simulink model "Two_D_Maps"  (R2020a)
settings: Solver=VariableStepAuto  StartTime=0.0  StopTime=inf  RelTol=1e-3
PostLoadFcn:
  | data1=xlsread('performancemaps','VE');
  | rpm1=data1(1,2:end);
  | map1=data1(2:end,1);
  | ve=data1(2:end,2:end);
  | 
  | data2=xlsread('performancemaps','Spark');
  | 
  | spark=data2(2:end,2:end);
  | 
  | data3=xlsread('performancemaps','AFR');
  | 
  | AFR=data3(2:end,2:end);
settings Model: Creator=sateeshk  LastModifiedBy=sateeshk

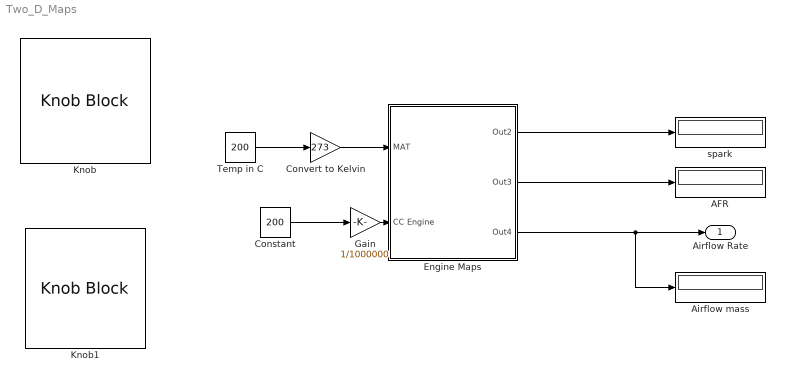
== system Two_D_Maps ==
  AFR : Display
  Airflow mass : Display
  Constant : Constant  Value=200
  Convert to Kelvin : Gain  Gain=273
  Engine Maps : Subsystem
  Gain : Gain  Gain=1/1000000
  Knob : KnobBlock  ScaleMin=1000  ScaleMax=10000
  Knob1 : KnobBlock  ScaleMin=25  ScaleMax=101
  Temp in C : Constant  Value=200
  spark : Display
  Airflow Rate : Outport
  wires:
  Engine Maps/1(Out2) -> spark/1
  Engine Maps/2(Out3) -> AFR/1
  Constant/1 -> Gain/1
  Gain/1 -> Engine Maps/2(CC Engine)
  Convert to Kelvin/1 -> Engine Maps/1(MAT)
  Temp in C/1 -> Convert to Kelvin/1
  Engine Maps/3(Out4) -> Airflow mass/1, Airflow Rate/1

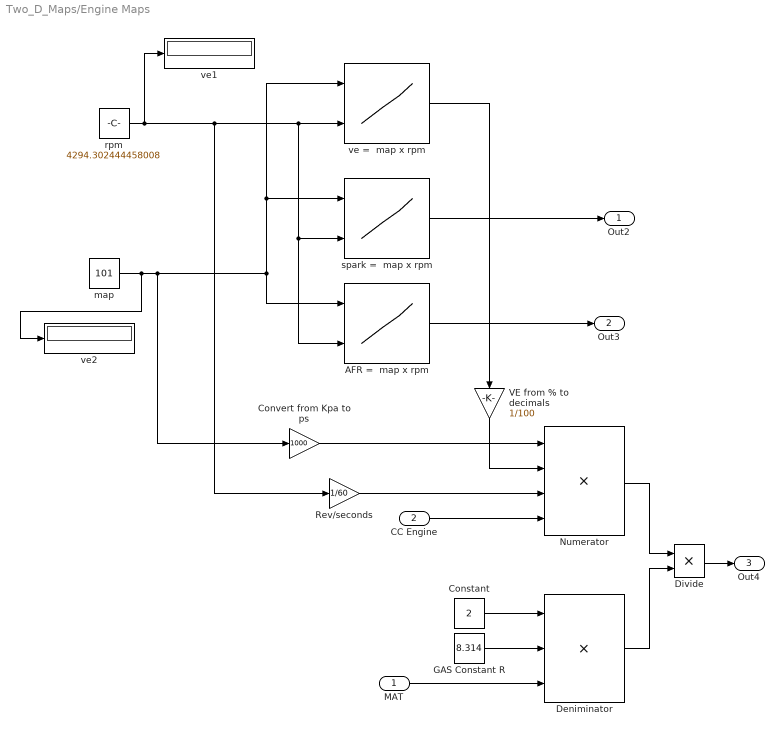
== system Two_D_Maps/Engine Maps ==
  MAT : Inport
  CC Engine : Inport  Port=2
  AFR =  map x rpm : Lookup_n-D  BreakpointsForDimension1=map1  BreakpointsForDimension2=rpm1  Table=AFR  InternalRulePriority=Speed  RndMeth=Simplest  InputSameDT=on
  Constant : Constant  Value=2
  Convert from Kpa to ps : Gain  Gain=1000
  Deniminator : Product  Inputs=***
  Divide : Product
  GAS Constant R : Constant  Value=8.314
  Numerator : Product  Inputs=****
  Rev/seconds : Gain  Gain=1/60
  VE from % to decimals : Gain  Gain=1/100
  map : Constant  Value=101
  rpm : Constant  Value=4294.302444458008
  spark =  map x rpm : Lookup_n-D  BreakpointsForDimension1=map1  BreakpointsForDimension2=rpm1  Table=spark  InternalRulePriority=Speed  RndMeth=Simplest  InputSameDT=on
  ve =  map x rpm : Lookup_n-D  BreakpointsForDimension1=map1  BreakpointsForDimension2=rpm1  Table=ve  InternalRulePriority=Speed  RndMeth=Simplest  InputSameDT=on
  ve1 : Display
  ve2 : Display
  Out2 : Outport
  Out3 : Outport  Port=2
  Out4 : Outport  Port=3
  wires:
  spark =  map x rpm/1 -> Out2/1
  ve =  map x rpm/1 -> VE from % to decimals/1
  AFR =  map x rpm/1 -> Out3/1
  map/1 -> ve2/1, Convert from Kpa to ps/1, ve =  map x rpm/1, spark =  map x rpm/1, AFR =  map x rpm/1
  rpm/1 -> Rev/seconds/1, AFR =  map x rpm/2, spark =  map x rpm/2, ve =  map x rpm/2, ve1/1
  Rev/seconds/1 -> Numerator/3
  Constant/1 -> Deniminator/1
  MAT/1 -> Deniminator/3
  GAS Constant R/1 -> Deniminator/2
  Numerator/1 -> Divide/1
  Deniminator/1 -> Divide/2
  Divide/1 -> Out4/1
  CC Engine/1 -> Numerator/4
  VE from % to decimals/1 -> Numerator/2
  Convert from Kpa to ps/1 -> Numerator/1
